simulink model "test_ppss_mdl"  (R2018b)
settings: Solver=VariableStepAuto  StartTime=0.0  StopTime=5  MaxStep=0.01  RelTol=1e-3  EnableMultiTasking=on
values from neighbouring files (symbols this model uses):
  pdG1 = pass(sys,[Zmin Zmax ; Mmin Mmax])    [test_lpvsyn.m]    (also in test_p_ss_subsref.m = pdG(idx1,idx2); test_pass.m = pass(a,b,c,d,setP,             'InputName','u','OutputName',; test_pass_interconnections.m = pass(a,b,c,d,pv,'InputName','u1','OutputName','y1'); test_pass_lft.m = pass(A,B,C,D,[0 2;2 6]))
libraries: cstblocks x1, simulink x1, lpvlibrary x1
settings Model: Creator=Fernando  LastModifiedBy=ferna
settings OptimizationCC: LifeSpan=inf
settings DebuggingCC: SFUnexpectedBacktrackingDiag=warning  SFNoUnconditionalDefaultTransitionDiag=warning
settings SFSimCC: SimUseLocalCustomCode=off
settings RTWCC: RTWUseLocalCustomCode=off
settings CodeAppCC: StateflowObjectComments=on
settings GRTTargetCC: TargetLangStandard=C89/C90 (ANSI)  GeneratePreprocessorConditionals=Disable all
settings ConfigComp: CovMetricSettings=dw  CovHtmlReporting=on  CovSaveCumulativeToWorkspaceVar=on  CovSaveSingleToWorkspaceVar=on  CovExternalEMLEnable=off

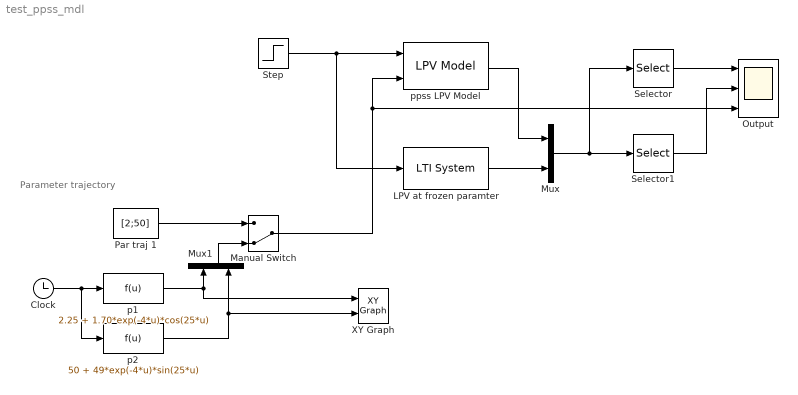
== system test_ppss_mdl ==
  note: Parameter trajectory
  Clock : Clock
  LPV at frozen paramter : cstblocks/LTI System  sys=ss(pdG1,[2;50])  IC=[]
  Manual Switch : ManualSwitch  CurrentSetting=0
  Mux : Mux  Inputs=2
  Mux1 : Mux  Inputs=2
  Output : Scope  NumInputPorts=3
  Par traj 1 : Constant  Value=[2;50]
  Selector : Selector  InputPortWidth=4  IndexOptions=Index vector (dialog)  Indices=[1 3]  OutputSizes=1
  Selector1 : Selector  InputPortWidth=4  IndexOptions=Index vector (dialog)  Indices=[2 4]  OutputSizes=1
  Step : Step  Time=0.2  SampleTime=0
  XY Graph : simulink/Sinks/XY Graph  xmin=0  xmax=5  ymin=0  ymax=110  st=-1
  p1 : Fcn  Expr=2.25 + 1.70*exp(-4*u)*cos(25*u)
  p2 : Fcn  Expr=50 + 49*exp(-4*u)*sin(25*u)
  ppss LPV Model : lpvlibrary/LPV Model  pdG=pdG1  x0=0
      settings: SourceProductName=LPV Toolbox
  wires:
  Clock/1 -> p2/1, p1/1
  p1/1 -> XY Graph/1, Mux1/1
  p2/1 -> Mux1/2, XY Graph/2
  Mux1/1 -> Manual Switch/2
  Par traj 1/1 -> Manual Switch/1
  ppss LPV Model/1 -> Mux/1
  Selector1/1 -> Output/2
  Selector/1 -> Output/1
  Mux/1 -> Selector/1, Selector1/1
  LPV at frozen paramter/1 -> Mux/2
  Step/1 -> ppss LPV Model/1, LPV at frozen paramter/1
  Manual Switch/1 -> ppss LPV Model/2, Output/3
